simulink model "rlModel"  (R2021b)
settings: Solver=VariableStepAuto  StartTime=0.0  StopTime=1000  RelTol=1e-3
libraries: rllib x6, deeplib x3
settings Model: Creator=Mitch  LastModifiedBy=Mitch

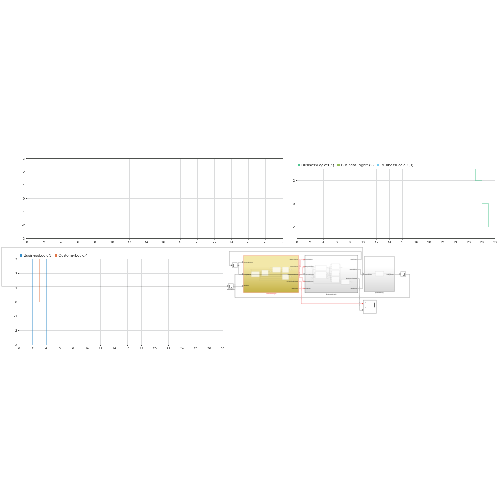
[thumbnail: Simulink's stored preview of the top-level diagram]
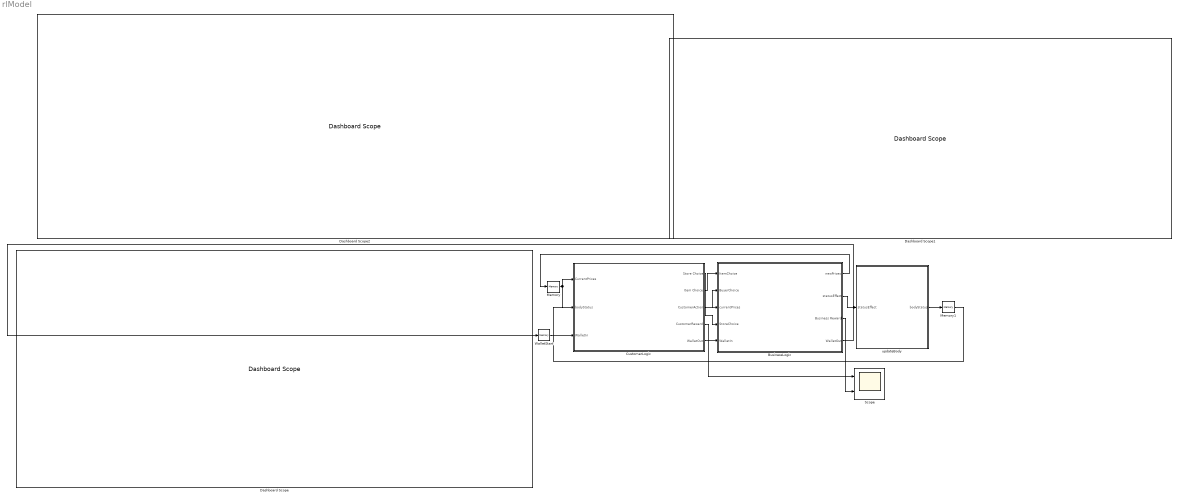
== system rlModel ==
  BusinessLogic : Subsystem
  CustomerLogic : Subsystem
  Dashboard Scope : DashboardScope
  Dashboard Scope1 : DashboardScope
  Dashboard Scope2 : DashboardScope
  Memory : Memory  InitialCondition=[50,50,50]
  Memory1 : Memory  InitialCondition=[100;100;100]
  Scope : Scope  NumInputPorts=2
  WalletStart : Memory  InitialCondition=500
  updateBody : Subsystem
  wires:
  CustomerLogic/3(CustomerAction) -> BusinessLogic/2(BuyerChoice)
  CustomerLogic/2(Item Choice) -> BusinessLogic/1(ItemChoice)
  BusinessLogic/2(statusEffect) -> updateBody/1(statusEffect)
  updateBody/1(bodyStatus) -> Memory1/1
  Memory1/1 -> CustomerLogic/2(bodyStatus)
  BusinessLogic/1(newPrices) -> Memory/1
  CustomerLogic/4(CustomerReward) -> Scope/1
  BusinessLogic/3(Business Reward) -> Scope/2
  CustomerLogic/1(Store Choice) -> BusinessLogic/4(StoreChoice)
  Memory/1 -> BusinessLogic/3(currentPrices), CustomerLogic/1(CurrentPrices)
  CustomerLogic/5(WalletOut) -> BusinessLogic/5(WalletIn)
  WalletStart/1 -> CustomerLogic/3(WalletIn)
  BusinessLogic/4(WalletOut) -> WalletStart/1

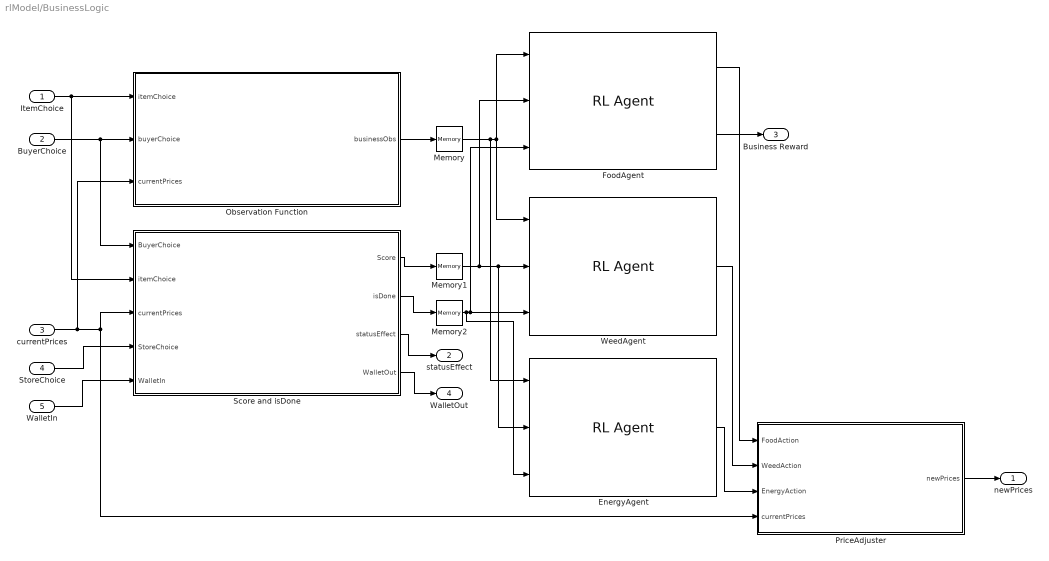
== system rlModel/BusinessLogic ==
  ItemChoice : Inport
  BuyerChoice : Inport  Port=2
  currentPrices : Inport  Port=3
  StoreChoice : Inport  Port=4
  WalletIn : Inport  Port=5
  EnergyAgent : rllib/RL Agent  Agent=EnergyAgent  ExternalActionAsInput=off  ProvideCumRwd=off  TreatAsDirectFeedthrough=on
  FoodAgent : rllib/RL Agent  Agent=FoodAgent  ExternalActionAsInput=off  ProvideCumRwd=on  TreatAsDirectFeedthrough=on
  Memory : Memory  InitialCondition=[0,0,0,0,0,0,0,0,0,0;0,0,0,0,0,0,0,0,0,0;0,0,0,0,0,0,0,0,0,0;0,0,0,0,0,0,0,0,0,0;0,0,0,0,0,0,0,0,0,0]
  Memory1 : Memory
  Memory2 : Memory
  Observation Function : MATLAB Function  TreatAsAtomicUnit=on
  PriceAdjuster : MATLAB Function  TreatAsAtomicUnit=on
  Score and isDone : Subsystem
  WeedAgent : rllib/RL Agent  Agent=WeedAgent  ExternalActionAsInput=off  ProvideCumRwd=off  TreatAsDirectFeedthrough=on
  newPrices : Outport
  statusEffect : Outport  Port=2
  Business Reward : Outport  Port=3
  WalletOut : Outport  Port=4
  wires:
  EnergyAgent/1 -> PriceAdjuster/3(EnergyAction)
  PriceAdjuster/1(newPrices) -> newPrices/1
  FoodAgent/2 -> Business Reward/1
  Observation Function/1(businessObs) -> Memory/1
  Score and isDone/2(isDone) -> Memory2/1
  Score and isDone/3(statusEffect) -> statusEffect/1
  currentPrices/1 -> Score and isDone/3(currentPrices), PriceAdjuster/4(currentPrices), Observation Function/3(currentPrices)
  WeedAgent/1 -> PriceAdjuster/2(WeedAction)
  BuyerChoice/1 -> Score and isDone/1(BuyerChoice), Observation Function/2(buyerChoice)
  FoodAgent/1 -> PriceAdjuster/1(FoodAction)
  StoreChoice/1 -> Score and isDone/4(StoreChoice)
  Score and isDone/1(Score) -> Memory1/1
  Memory2/1 -> WeedAgent/3, FoodAgent/3, EnergyAgent/3
  Memory1/1 -> EnergyAgent/2, WeedAgent/2, FoodAgent/2
  Memory/1 -> FoodAgent/1, WeedAgent/1, EnergyAgent/1
  ItemChoice/1 -> Score and isDone/2(itemChoice), Observation Function/1(itemChoice)
  WalletIn/1 -> Score and isDone/5(WalletIn)
  Score and isDone/4(WalletOut) -> WalletOut/1

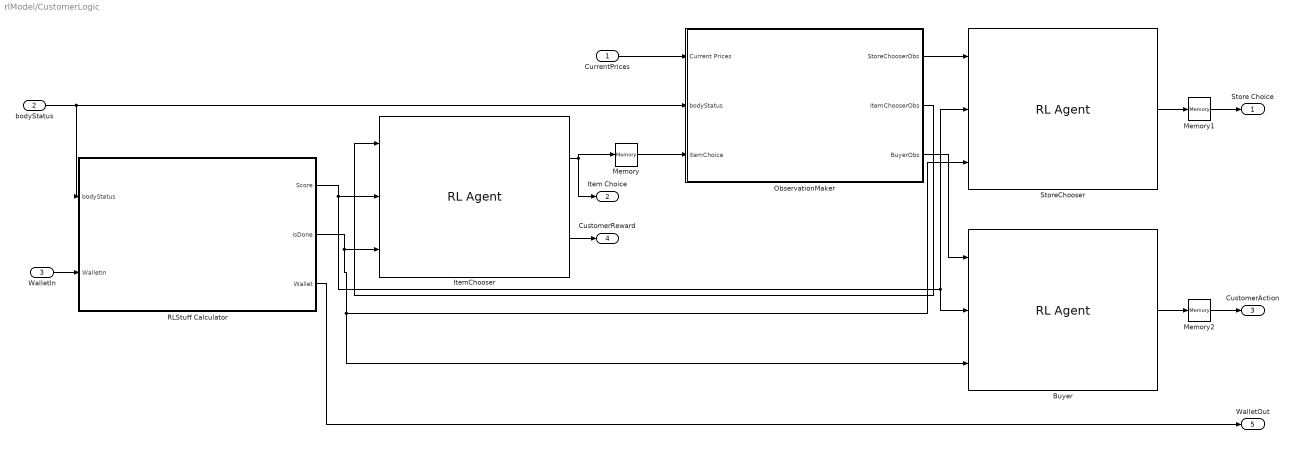
== system rlModel/CustomerLogic ==
  CurrentPrices : Inport
  bodyStatus : Inport  Port=2
  WalletIn : Inport  Port=3
  Buyer : rllib/RL Agent  Agent=Buyer  ExternalActionAsInput=off  ProvideCumRwd=off  TreatAsDirectFeedthrough=on
  ItemChooser : rllib/RL Agent  Agent=ItemChooser  ExternalActionAsInput=off  ProvideCumRwd=on  TreatAsDirectFeedthrough=on
  Memory : Memory  InitialCondition=1
  Memory1 : Memory  InitialCondition=1
  Memory2 : Memory  InitialCondition=1
  ObservationMaker : Subsystem
  RLStuff Calculator : Subsystem
  StoreChooser : rllib/RL Agent  Agent=StoreChooser  ExternalActionAsInput=off  ProvideCumRwd=off  TreatAsDirectFeedthrough=on
  Store Choice : Outport
  Item Choice : Outport  Port=2
  CustomerAction : Outport  Port=3
  CustomerReward : Outport  Port=4
  WalletOut : Outport  Port=5
  wires:
  ItemChooser/2 -> CustomerReward/1
  Memory1/1 -> Store Choice/1
  Memory2/1 -> CustomerAction/1
  Memory/1 -> ObservationMaker/3(itemChoice)
  ObservationMaker/2(ItemChooserObs) -> ItemChooser/1
  ObservationMaker/3(BuyerObs) -> Buyer/1
  StoreChooser/1 -> Memory1/1
  ItemChooser/1 -> Item Choice/1, Memory/1
  ObservationMaker/1(StoreChooserObs) -> StoreChooser/1
  Buyer/1 -> Memory2/1
  CurrentPrices/1 -> ObservationMaker/1(Current Prices)
  RLStuff Calculator/1(Score) -> StoreChooser/2, Buyer/2, ItemChooser/2
  RLStuff Calculator/2(isDone) -> StoreChooser/3, Buyer/3, ItemChooser/3
  bodyStatus/1 -> ObservationMaker/2(bodyStatus), RLStuff Calculator/1(bodyStatus)
  RLStuff Calculator/3(Wallet) -> WalletOut/1
  WalletIn/1 -> RLStuff Calculator/2(WalletIn)

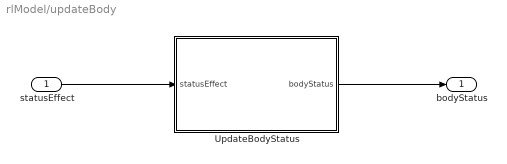
== system rlModel/updateBody ==
  statusEffect : Inport
  UpdateBodyStatus : MATLAB Function  TreatAsAtomicUnit=on
  bodyStatus : Outport
  wires:
  UpdateBodyStatus/1(bodyStatus) -> bodyStatus/1
  statusEffect/1 -> UpdateBodyStatus/1(statusEffect)

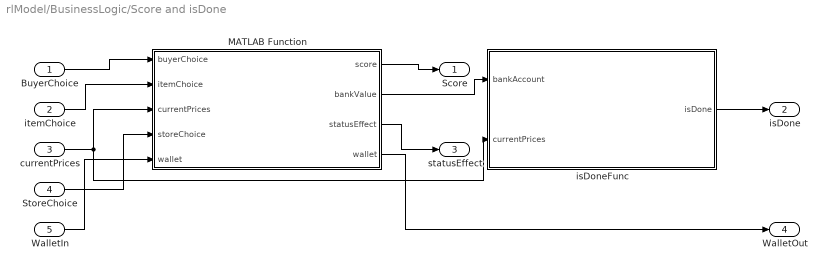
== system rlModel/BusinessLogic/Score and isDone ==
  BuyerChoice : Inport
  itemChoice : Inport  Port=2
  currentPrices : Inport  Port=3
  StoreChoice : Inport  Port=4
  WalletIn : Inport  Port=5
  MATLAB Function : MATLAB Function  TreatAsAtomicUnit=on
  isDoneFunc : MATLAB Function  TreatAsAtomicUnit=on
  Score : Outport
  isDone : Outport  Port=2
  statusEffect : Outport  Port=3
  WalletOut : Outport  Port=4
  wires:
  BuyerChoice/1 -> MATLAB Function/1(buyerChoice)
  itemChoice/1 -> MATLAB Function/2(itemChoice)
  currentPrices/1 -> isDoneFunc/2(currentPrices), MATLAB Function/3(currentPrices)
  MATLAB Function/1(score) -> Score/1
  MATLAB Function/2(bankValue) -> isDoneFunc/1(bankAccount)
  MATLAB Function/3(statusEffect) -> statusEffect/1
  isDoneFunc/1(isDone) -> isDone/1
  StoreChoice/1 -> MATLAB Function/4(storeChoice)
  MATLAB Function/4(wallet) -> WalletOut/1
  WalletIn/1 -> MATLAB Function/5("wallet ")

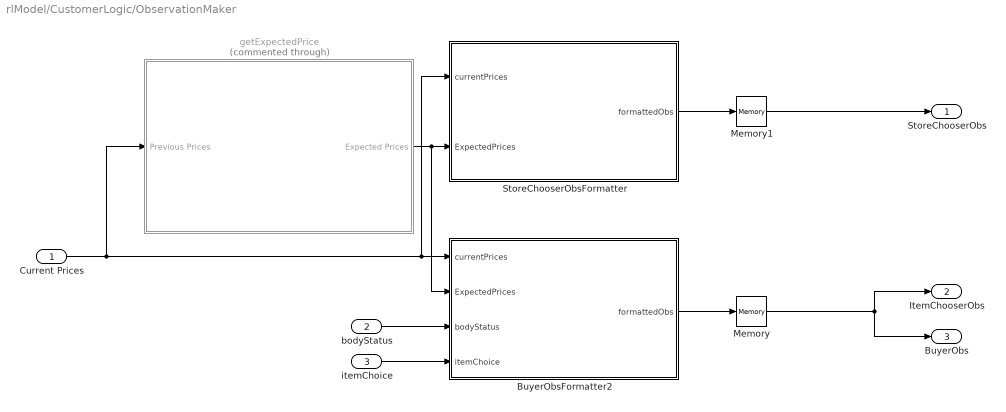
== system rlModel/CustomerLogic/ObservationMaker ==
  Current Prices : Inport
  bodyStatus : Inport  Port=2
  itemChoice : Inport  Port=3
  BuyerObsFormatter2 : MATLAB Function  TreatAsAtomicUnit=on
  Memory : Memory  InitialCondition=[0,0,0,0,0,0,0,0,0,0;0,0,0,0,0,0,0,0,0,0;0,0,0,0,0,0,0,0,0,0;0,0,0,0,0,0,0,0,0,0;0,0,0,0,0,0,0,0,0,0;0,0,0,0,0,0,0,0,0,0;0,0,0,0,0,0,0,0,0,0;0,0,0,0,0,0,0,0,0,0;0,0,0,0,0,0,0,0,0,0;0,0,0,0,0,0,0,0,0,0;]
  Memory1 : Memory  InitialCondition=[0,0,0,0,0,0,0,0,0,0;0,0,0,0,0,0,0,0,0,0;0,0,0,0,0,0,0,0,0,0;0,0,0,0,0,0,0,0,0,0;0,0,0,0,0,0,0,0,0,0;0,0,0,0,0,0,0,0,0,0;]
  StoreChooserObsFormatter : MATLAB Function  TreatAsAtomicUnit=on
  getExpectedPrice : Subsystem  Commented=through
  StoreChooserObs : Outport
  ItemChooserObs : Outport  Port=2
  BuyerObs : Outport  Port=3
  wires:
  itemChoice/1 -> BuyerObsFormatter2/4(itemChoice)
  bodyStatus/1 -> BuyerObsFormatter2/3(bodyStatus)
  Current Prices/1 -> BuyerObsFormatter2/1(currentPrices), StoreChooserObsFormatter/1(currentPrices), getExpectedPrice/1(Previous Prices)
  getExpectedPrice/1(Expected Prices) -> BuyerObsFormatter2/2(ExpectedPrices), StoreChooserObsFormatter/2(ExpectedPrices)
  Memory/1 -> ItemChooserObs/1, BuyerObs/1
  BuyerObsFormatter2/1(formattedObs) -> Memory/1
  StoreChooserObsFormatter/1(formattedObs) -> Memory1/1
  Memory1/1 -> StoreChooserObs/1

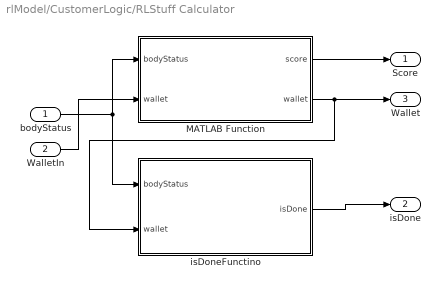
== system rlModel/CustomerLogic/RLStuff Calculator ==
  bodyStatus : Inport
  WalletIn : Inport  Port=2
  MATLAB Function : MATLAB Function  TreatAsAtomicUnit=on
  isDoneFunctino : MATLAB Function  TreatAsAtomicUnit=on
  Score : Outport
  isDone : Outport  Port=2
  Wallet : Outport  Port=3
  wires:
  isDoneFunctino/1(isDone) -> isDone/1
  bodyStatus/1 -> MATLAB Function/1(bodyStatus), isDoneFunctino/1(bodyStatus)
  MATLAB Function/1(score) -> Score/1
  MATLAB Function/2(wallet) -> Wallet/1, isDoneFunctino/2(wallet)
  WalletIn/1 -> MATLAB Function/2("wallet ")

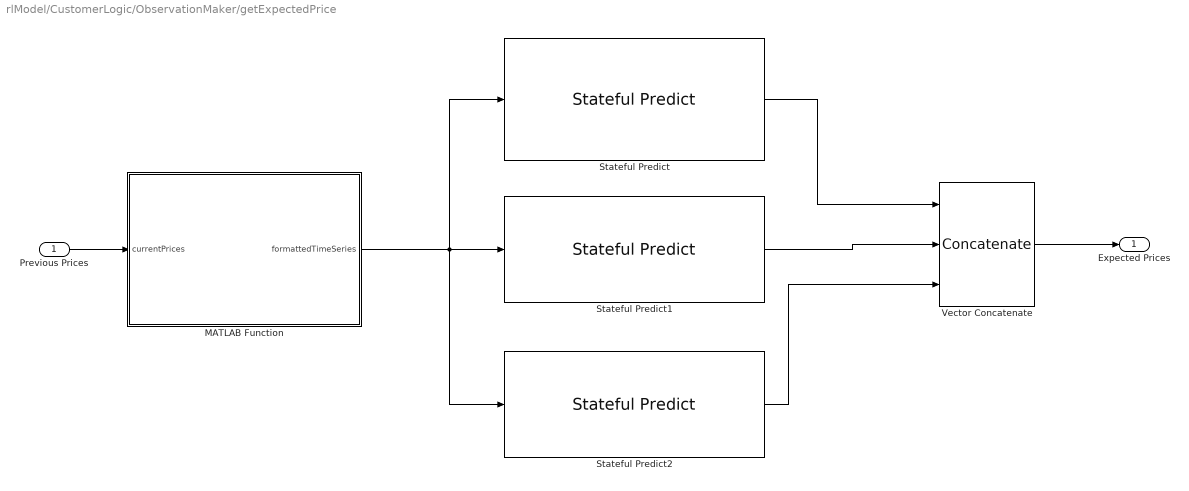
== system rlModel/CustomerLogic/ObservationMaker/getExpectedPrice ==
  Previous Prices : Inport
  MATLAB Function : MATLAB Function  TreatAsAtomicUnit=on
  Stateful Predict : deeplib/Stateful Predict  Network=Network from MAT-file  NetworkFunction=untitled  NetworkFilePath=foodNet.mat  InputDataFormats={'',''}  SampleTime=-1  ForceInterpretedSim=off  EnableDLNetwork=on
      settings: SourceProductBaseCode=NN
  Stateful Predict1 : deeplib/Stateful Predict  Network=Network from MAT-file  NetworkFunction=untitled  NetworkFilePath=drugsNet.mat  InputDataFormats={ '', '' }  SampleTime=-1  ForceInterpretedSim=off  EnableDLNetwork=on
      settings: SourceProductBaseCode=NN
  Stateful Predict2 : deeplib/Stateful Predict  Network=Network from MAT-file  NetworkFunction=untitled  NetworkFilePath=energyDrinkNet.mat  InputDataFormats={ '', '' }  SampleTime=-1  ForceInterpretedSim=off  EnableDLNetwork=on
      settings: SourceProductBaseCode=NN
  Vector Concatenate : Concatenate  NumInputs=3
  Expected Prices : Outport
  wires:
  Previous Prices/1 -> MATLAB Function/1(currentPrices)
  MATLAB Function/1(formattedTimeSeries) -> Stateful Predict/1, Stateful Predict2/1, Stateful Predict1/1
  Vector Concatenate/1 -> Expected Prices/1
  Stateful Predict/1 -> Vector Concatenate/1
  Stateful Predict2/1 -> Vector Concatenate/3
  Stateful Predict1/1 -> Vector Concatenate/2

== matlab function rlModel/CustomerLogic/ObservationMaker/getExpectedPrice/MATLAB Function ==
  data: currentPrices input; formattedTimeSeries output
function formattedTimeSeries  = formatInputSeq(currentPrices)

numFeatures = length(currentPrices);
timeSteps = 5;

%Setup Persistent Variables
persistent oldPrices; 

if(isempty(oldPrices))
     oldPrices = zeros(numFeatures, timeSteps);
end

if(size(currentPrices, 2) > 1)
    currentPrices = currentPrices';
end
    
%Concatinate all but one of the old prices
formattedTimeSeries = [oldPrices(:, 2:end), currentPrices];

oldPrices = formattedTimeSeries;

== matlab function rlModel/CustomerLogic/ObservationMaker/StoreChooserObsFormatter ==
  data: currentPrices input; formattedObs output; ExpectedPrices input
function formattedObs = buyerObsMaker(currentPrices, ExpectedPrices)

timeSteps = 10;

newObservation = [currentPrices; ExpectedPrices];

persistent oldObservations

formattedObs = zeros(6, timeSteps);

if(isempty(oldObservations))
     oldObservations = zeros(6, timeSteps);
end


formattedObs = [oldObservations(:, 2:end), newObservation];

oldObservations = formattedObs;

== matlab function rlModel/CustomerLogic/RLStuff Calculator/isDoneFunctino ==
  data: bodyStatus input; isDone output; wallet input
function isDone = isDoneStatus(bodyStatus, wallet)
%Put all the end conditions here
%
% Death:
%   -Starvation
%   -exhaustion
%   -boredom

%Basic Death Functions
if(bodyStatus(1) == 0)
    fprintf("\nDied of Starvation!")
    isDone = 1;
elseif(bodyStatus(2) == 0)
    fprintf("\nDied of exhaustion!")
    isDone = 1;
elseif(bodyStatus(3) == 0)
    fprintf("\nDied of boredom!")
    isDone = 1;
else
    isDone = 0;
end

%Wallet
if(wallet <= 0)
   isDone = 1;
end

== matlab function rlModel/CustomerLogic/ObservationMaker/BuyerObsFormatter2 ==
  data: currentPrices input; formattedObs output; ExpectedPrices input; bodyStatus input; itemChoice input
function formattedObs = buyerObsMaker(currentPrices, ExpectedPrices, bodyStatus, itemChoice)

timeSteps = 10;

newObservation = [currentPrices', ExpectedPrices', bodyStatus', itemChoice]';

persistent oldObservations

if(isempty(oldObservations))
     oldObservations = zeros(10, timeSteps);
end

formattedObs = [oldObservations(:, 2:end), newObservation];

oldObservations = formattedObs;

== matlab function rlModel/CustomerLogic/RLStuff Calculator/MATLAB Function ==
  data: bodyStatus input; score output; wallet input; wallet output
function [score, wallet] = fcn(bodyStatus, wallet)
score = 0;

persistent oldStatus
if(isempty(oldStatus))
    oldStatus = zeros(3, 1);
end

%Assume they have a job
wallet = wallet + 30;

change = bodyStatus - oldStatus;

% stomach = bodyStatus(1);
% energy = bodyStatus(2);
% entertian = bodyStatus(3);

oldStatus = bodyStatus;

%Basics
%stomach
if(bodyStatus(1) > 100)
    score = score + 10;
else
    score = score - 5;
end

%energy
if(bodyStatus(2) > 100)
    score = score + 10;
else
    score = score - 5;
end

%Entertain 
if(bodyStatus(3) > 100)
    score = score + 10;
else
    score = score - 5;
end

%Wallet
if(wallet <= 0)
   score = score - 10;
end


%\Basics









end

== matlab function rlModel/updateBody/UpdateBodyStatus ==
  data: statusEffect input; bodyStatus output
function bodyStatus = fcn(statusEffect)

persistent oldBodyStatus

if(isempty(oldBodyStatus))
     oldBodyStatus = 100 * ones(3,1);
end

bodyStatus = oldBodyStatus + statusEffect;

oldBodyStatus = bodyStatus;

== matlab function rlModel/BusinessLogic/Observation Function ==
  data: businessObs output; itemChoice input; buyerChoice input; currentPrices input
function businessObs = makeBusinessObs(itemChoice, buyerChoice, currentPrices)

timeSteps = 10;

businessObs = zeros(5, timeSteps);

persistent oldbusinessObs

currentObs = [currentPrices', itemChoice, buyerChoice]';

if(isempty(oldbusinessObs))
    oldbusinessObs = zeros(5, timeSteps); 
end

if(size(currentObs, 2) > 1)
    businessObs = [oldbusinessObs(:, 2:end), currentObs'];
else
    businessObs = [oldbusinessObs(:, 2:end), currentObs];
end

oldbusinessObs = businessObs;

== matlab function rlModel/BusinessLogic/Score and isDone/MATLAB Function ==
  data: score output; buyerChoice input; itemChoice input; currentPrices input; bankValue output; statusEffect output; storeChoice input; wallet input; wallet output
function [score, bankValue, statusEffect, wallet] = fcn(buyerChoice, itemChoice, currentPrices, storeChoice, wallet)

score = 0;

storeNum = 1;

persistent bankAccount;

if(isempty(bankAccount))
   bankAccount = 500; 
end

% items = ["Food", "Weed", "EnergyDrink"];
itemPrices      = [25,40,3];
possibleEffects = [[3, -1, 0]', [0, 3, -1]' [-1, 0, 3]'];

statusEffect = possibleEffects(:, itemChoice);

expenses = (buyerChoice * (itemPrices(itemChoice)));
revenue = (buyerChoice * (currentPrices(itemChoice)));
profit = revenue - expenses;

wallet = wallet - revenue;

bankAccount = bankAccount + profit;

if(storeChoice ~= storeNum)
    score = score - 20;
    profit = 0;
end

if(profit == 0)
    score = score - 5;
elseif(profit > 0)
    score = score + 10;
else
    score = score - 10;
end

bankValue = bankAccount;
    
end

== matlab function rlModel/BusinessLogic/PriceAdjuster ==
  data: FoodAction input; newPrices output; WeedAction input; EnergyAction input; currentPrices input
function newPrices = fcn(FoodAction, WeedAction, EnergyAction, currentPrices)

amount = 2;

%Food price either increases or decreases
if(FoodAction == 1)
    currentPrices(1) = currentPrices(1) - amount;
else
    currentPrices(1) = currentPrices(1) + amount;
end

if(WeedAction == 1)
    currentPrices(2) = currentPrices(2) - amount;
else
    currentPrices(2) = currentPrices(2) + amount;
end

if(EnergyAction == 1)
    currentPrices(3) = currentPrices(3) - amount;
else
    currentPrices(3) = currentPrices(3) + amount;
end

newPrices = [currentPrices];


end

== matlab function rlModel/BusinessLogic/Score and isDone/isDoneFunc ==
  data: isDone output; bankAccount input; currentPrices input
function isDone = fcn(bankAccount, currentPrices)

isDone = 0;

if(bankAccount <= 0)
    isDone = 1;
end

A = (currentPrices <= 0);

if(sum(A) >= 1)
    isDone = 1;
end

end
